simulink model "model"  (R2020b)
settings: Solver=VariableStepAuto  StartTime=0.0  StopTime=180.0  RelTol=1e-3
values from neighbouring files (symbols this model uses):
  a_phi1 = 2.87    [Problem2.m]
  a_phi2 = -0.65    [Problem2.m]
  d = 1.5*deg2rad    (= 0.0261799387799)    [Problem2.m]
  g = 9.81    [Problem2.m]    (also in bank_to_turn.m)
  k_dphi = (2*zeta_phi*omega_nphi-a_phi1)/a_phi2    [Problem2.m]
  k_ichi = (omega_nchi^2*V_g)/g    [Problem2.m]
  k_pchi = (2*zeta_chi*omega_nchi*V_g)/g    [Problem2.m]
  k_pphi = -2    [Problem2.m]
  V_g = 580    [Problem2.m]    (also in bank_to_turn.m)
settings Model: Creator=ingridnorland  LastModifiedBy=ingridnorland

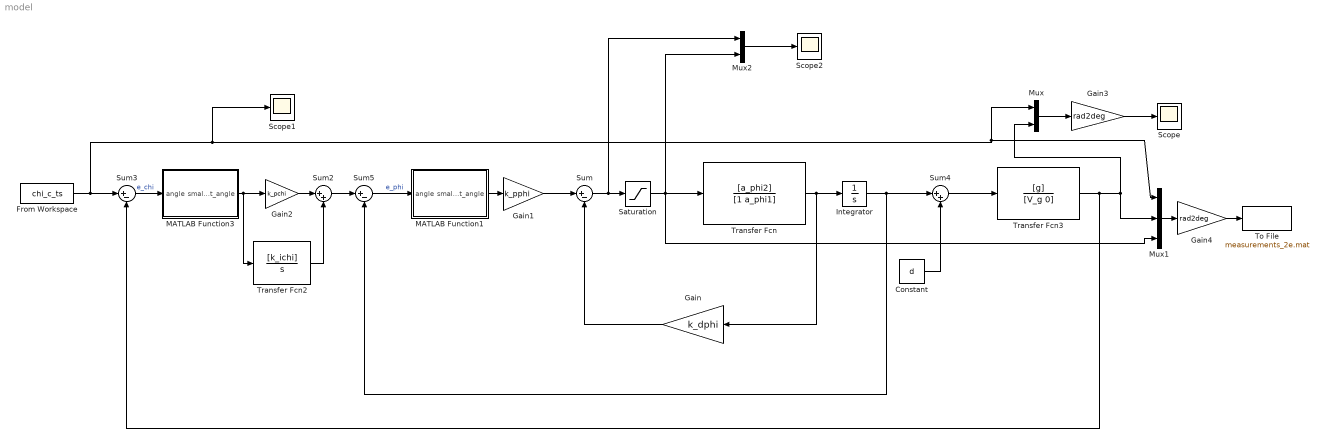
== system model ==
  Constant : Constant  Value=d
  From Workspace : FromWorkspace  VariableName=chi_c_ts
  Gain : Gain  Gain=k_dphi
  Gain1 : Gain  Gain=k_pphi
  Gain2 : Gain  Gain=k_pchi
  Gain3 : Gain  Gain=rad2deg
  Gain4 : Gain  Gain=rad2deg
  Integrator : Integrator
  MATLAB Function1 : MATLAB Function  TreatAsAtomicUnit=on
  MATLAB Function3 : MATLAB Function  TreatAsAtomicUnit=on
  Mux : Mux  Inputs=2
  Mux1 : Mux  Inputs=3
  Mux2 : Mux  Inputs=2
  Saturation : Saturate  UpperLimit=30*deg2rad  LowerLimit=-30*deg2rad
  Scope : Scope
  Scope1 : Scope
  Scope2 : Scope
  Sum : Sum  Inputs=|+-
  Sum2 : Sum  Inputs=|++
  Sum3 : Sum  Inputs=|+-
  Sum4 : Sum  Inputs=|++
  Sum5 : Sum  Inputs=|+-
  To File : ToFile  Filename=measurements_2e.mat  MatrixName=measurements
  Transfer Fcn : TransferFcn  Numerator=[a_phi2]  Denominator=[1 a_phi1]
  Transfer Fcn2 : TransferFcn  Numerator=[k_ichi]  Denominator=[1 0]
  Transfer Fcn3 : TransferFcn  Numerator=[g]  Denominator=[V_g 0]
  wires:
  Transfer Fcn/1 -> Gain/1, Integrator/1
  Gain/1 -> Sum/2
  Gain1/1 -> Sum/1
  Gain2/1 -> Sum2/1
  Transfer Fcn2/1 -> Sum2/2
  Constant/1 -> Sum4/2
  Sum4/1 -> Transfer Fcn3/1
  Integrator/1 -> Sum4/1, Sum5/2
  Sum2/1 -> Sum5/1
  From Workspace/1 -> Mux/1, Mux1/1, Scope1/1, Sum3/1
  Transfer Fcn3/1 -> Mux/2, Mux1/2, Sum3/2
  Mux/1 -> Gain3/1
  Mux1/1 -> Gain4/1
  Gain4/1 -> To File/1
  Gain3/1 -> Scope/1
  Sum/1 -> Saturation/1, Mux2/1
  Sum3/1 -> MATLAB Function3/1(angle)  "e_chi"
  MATLAB Function3/1(smallest_angle) -> Transfer Fcn2/1, Gain2/1
  MATLAB Function1/1(smallest_angle) -> Gain1/1
  Sum5/1 -> MATLAB Function1/1(angle)  "e_phi"
  Saturation/1 -> Mux2/2, Mux1/3, Transfer Fcn/1
  Mux2/1 -> Scope2/1

== matlab function model/MATLAB Function3 ==
  data: angle input; smallest_angle output
function smallest_angle = my_ssa(angle)

smallest_angle = ssa(angle,'rad');

== matlab function model/MATLAB Function1 ==
  data: angle input; smallest_angle output
function smallest_angle = my_ssa(angle)

smallest_angle = ssa(angle,'rad');
